simulink model "lunar_lander_sim_mi"  (R2023a)
settings: Solver=VariableStepAuto  StartTime=0.0  StopTime=10  RelTol=1e-3
values from neighbouring files (symbols this model uses):
  D = 0:0.01:0.9    [limit_cycle_est.m]
undefined symbols (not defined in the file or in its folder): aMode
libraries: sharedutil x1, slpidlib x1
settings Model: Creator=s3928  LastModifiedBy=cnsl

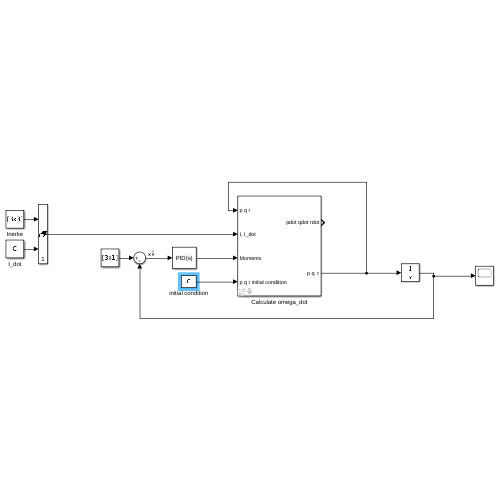
[thumbnail: Simulink's stored preview of the top-level diagram]
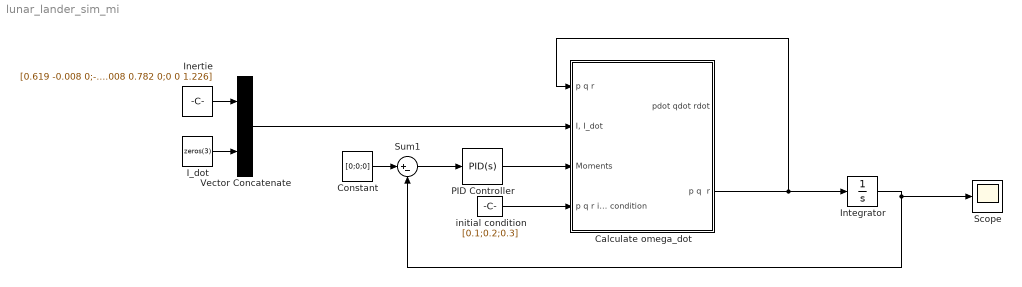
== system lunar_lander_sim_mi ==
  Calculate omega_dot : Subsystem  AncestorBlock=shared6dofsys/Calculate omega_dot  mask{aMode=aMode}
      mask init:
      | if aerosharedtest(gcb)
      |     aerosharedicon('shared');
      | else
      |     sharedautoicon('shared');
      | end
      settings: LibrarySourceBlock=shared6dofsys/Calculate omega_dot
  Constant : Constant  Value=[0;0;0]
  I_dot : Constant  Value=zeros(3)
  Inertie : Constant  Value=[0.619 -0.008 0;-0.008 0.782 0;0 0 1.226]
  Integrator : Integrator
  PID Controller : slpidlib/PID Controller  Controller=PID  Form=Parallel  TimeDomain=Continuous-time  UseExternalTs=off  SampleTime=-1  IntegratorMethod=Forward Euler  FilterMethod=Forward Euler  ControllerParametersSource=internal  P=10  I=10  UseKiTs=off  D=10  N=100  UseFilter=on  TunerSelectOption=Transfer Function Based (PID Tuner App)  InitialConditionSource=internal  InitialConditionForIntegrator=0  InitialConditionForFilter=0  DifferentiatorICPrevScaledInput=0  ExternalReset=none  TrackingMode=off  Kt=1  LimitOutput=off  SatLimitsSource=internal  UpperSaturationLimit=inf  LowerSaturationLimit=-inf  LinearizeAsGain=on  AntiWindupMode=none  Kb=1  LimitIntegrator=off  UpperIntegratorSaturationLimit=inf  LowerIntegratorSaturationLimit=-inf  POutMin=[]  POutMax=[]  IOutMin=[]  IOutMax=[]  DOutMin=[]  DOutMax=[]  NOutMin=[]  NOutMax=[]  SumOutMin=[]  SumOutMax=[]  SaturationOutMin=[]  SaturationOutMax=[]  PParamMin=[]  PParamMax=[]  IParamMin=[]  IParamMax=[]  DParamMin=[]  DParamMax=[]  NParamMin=[]  NParamMax=[]  KbParamMin=[]  KbParamMax=[]  KtParamMin=[]  KtParamMax=[]  KbOutMin=[]  KbOutMax=[]  KtOutMin=[]  KtOutMax=[]  IntegratorOutMin=[]  IntegratorOutMax=[]  FilterOutMin=[]  FilterOutMax=[]  SumI1OutMin=[]  SumI1OutMax=[]  SumI2OutMin=[]  SumI2OutMax=[]  SumI3OutMin=[]  SumI3OutMax=[]  SumI4OutMin=[]  SumI4OutMax=[]  SumDOutMin=[]  SumDOutMax=[]  DifferentiatorOutMin=[]  DifferentiatorOutMax=[]  FilterDiffOutCoefMin=[]  FilterDiffOutCoefMax=[]  ReciprocalOutMin=[]  ReciprocalOutMax=[]  SumDenOutMin=[]  SumDenOutMax=[]  SumNumOutMin=[]  SumNumOutMax=[]  DivideOutMin=[]  DivideOutMax=[]  UdiffTsProdOutMin=[]  UdiffTsProdOutMax=[]  NTsProdOutMin=[]  NTsProdOutMax=[]  UintegralTsProdOutMin=[]  UintegralTsProdOutMax=[]  UngainTsProdOutMin=[]  UngainTsProdOutMax=[]  ClampingZeroOutDataTypeStr=Inherit: Inherit via back propagation  ClampingZeroOutMin=[]  ClampingZeroOutMax=[]  FilterDenConstantOutDataTypeStr=Inherit: Inherit via back propagation  FilterDenConstantOutMin=[]  FilterDenConstantOutMax=[]  PCopyOutDataTypeStr=Inherit: Inherit via back propagation  PCopyOutMin=[]  PCopyOutMax=[]  NCopyOutDataTypeStr=Inherit: Inherit via back propagation  NCopyOutMin=[]  NCopyOutMax=[]  IntegratorContinuousStateAttributes=''  IntegratorStateMustResolveToSignalObject=off  IntegratorRTWStateStorageClass=Auto  FilterContinuousStateAttributes=''  FilterStateMustResolveToSignalObject=off  FilterRTWStateStorageClass=Auto  ParallelPVariant=InternalParameters  IdealPVariant=Disabled  IVariant=InternalParameters  DVariant=InternalParameters  IntegratorVariant=Continuous  SatVariant=Disabled  AWVariant=Passthrough  PCopyVariant=Disabled  TRVariant=Disabled  FdbkBlocksVariant=Forward  IdealPFdbkVariant=Disabled  SatFdbkVariant=Disabled  DerivativeFilterVariant=ContFilter  NVariant=InternalParameters  NCopyVariant=Disabled  FilterICVariant=InternalICsFilter  IntegratorICVariant=InternalICs  ExternalResetVariant=Disabled  TRSumVariant=Passthrough  SumFdbkVariant=Disabled  SumVariant=Sum_PID  TsampFilterVariant=InternalTs  TsampNgainVariant=Passthrough  TsampIntegralVariant=Disabled_SignalSpec  ExternalSaturationOutDataTypeStr=Inherit: Same as second input
  Scope : Scope
  Sum1 : Sum  Inputs=|+-
  Vector Concatenate : Concatenate  Mode=Multidimensional array
  initial condition : Constant  Value=[0.1;0.2;0.3]
  wires:
  Inertie/1 -> Vector Concatenate/1
  I_dot/1 -> Vector Concatenate/2
  Vector Concatenate/1 -> Calculate omega_dot/2("I, I_dot")
  Sum1/1 -> PID Controller/1
  Constant/1 -> Sum1/1
  Calculate omega_dot/2(p q  r) -> Integrator/1, Calculate omega_dot/1(p q r)
  initial condition/1 -> Calculate omega_dot/4(p q r initial condition)
  Integrator/1 -> Scope/1, Sum1/2
  PID Controller/1 -> Calculate omega_dot/3(Moments)

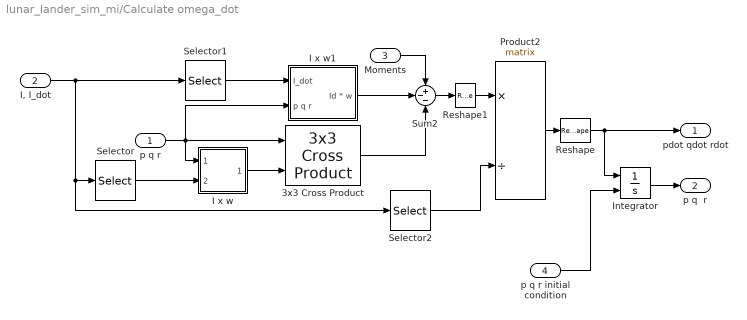
== system lunar_lander_sim_mi/Calculate omega_dot ==
  p q r : Inport  OutDataTypeStr=double
  "I, I_dot" : Inport  Port=2  OutDataTypeStr=double
  Moments : Inport  Port=3  OutDataTypeStr=double
  p q r initial condition : Inport  Port=4
  3x3 Cross Product : sharedutil/3x3 Cross Product  aMode=aMode
  I x w : Subsystem
  I x w1 : Subsystem
  Integrator : Integrator  InitialConditionSource=external
  Product2 : Product  Inputs=*/  Multiplication=Matrix(*)  SaturateOnIntegerOverflow=on  OutDataTypeStr=Inherit: Same as first input
  Reshape : Reshape
  Reshape1 : Reshape  OutputDimensionality=Row vector (2-D)
  Selector : Selector  NumberOfDimensions=2  InputPortWidth=2  IndexOptions=Index vector (dialog),Select all  Indices=1:3,-1  OutputSizes=1
  Selector1 : Selector  NumberOfDimensions=2  InputPortWidth=2  IndexOptions=Index vector (dialog),Select all  Indices=4:6,-1  OutputSizes=1
  Selector2 : Selector  NumberOfDimensions=2  InputPortWidth=2  IndexOptions=Index vector (dialog),Select all  Indices=1:3,-1  OutputSizes=1
  Sum2 : Sum  Inputs=+--  SaturateOnIntegerOverflow=on
  pdot qdot rdot : Outport  OutDataTypeStr=double  VectorParamsAs1DForOutWhenUnconnected=off
  p q  r : Outport  Port=2
  wires:
  Reshape1/1 -> Product2/1
  I x w/1(I * w) -> 3x3 Cross Product/2
  3x3 Cross Product/1 -> Sum2/3
  Selector1/1 -> I x w1/1(I_dot)
  I x w1/1(Id * w) -> Sum2/2
  Moments/1 -> Sum2/1
  Sum2/1 -> Reshape1/1
  Product2/1 -> Reshape/1
  p q r/1 -> I x w/1(p q r), I x w1/2(p q r), 3x3 Cross Product/1
  "I, I_dot"/1 -> Selector1/1, Selector2/1, Selector/1
  Selector2/1 -> Product2/2
  Selector/1 -> I x w/2(Inertia)
  Reshape/1 -> Integrator/1, pdot qdot rdot/1
  Integrator/1 -> p q  r/1
  p q r initial condition/1 -> Integrator/2

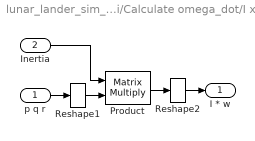
== system lunar_lander_sim_mi/Calculate omega_dot/I x w ==
  p q r : Inport
  Inertia : Inport  Port=2
  Product : Product  Multiplication=Matrix(*)  InputSameDT=on  SaturateOnIntegerOverflow=on  OutDataTypeStr=Inherit: Same as first input
  Reshape1 : Reshape  OutputDimensionality=Column vector (2-D)
  Reshape2 : Reshape
  I * w : Outport  VectorParamsAs1DForOutWhenUnconnected=off
  wires:
  Reshape2/1 -> I * w/1
  Reshape1/1 -> Product/2
  p q r/1 -> Reshape1/1
  Inertia/1 -> Product/1
  Product/1 -> Reshape2/1

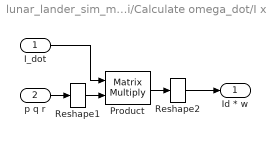
== system lunar_lander_sim_mi/Calculate omega_dot/I x w1 ==
  I_dot : Inport
  p q r : Inport  Port=2
  Product : Product  Multiplication=Matrix(*)  InputSameDT=on  SaturateOnIntegerOverflow=on  OutDataTypeStr=Inherit: Same as first input
  Reshape1 : Reshape  OutputDimensionality=Column vector (2-D)
  Reshape2 : Reshape
  Id * w : Outport  VectorParamsAs1DForOutWhenUnconnected=off
  wires:
  Reshape2/1 -> Id * w/1
  Reshape1/1 -> Product/2
  Product/1 -> Reshape2/1
  I_dot/1 -> Product/1
  p q r/1 -> Reshape1/1
